simulink model "driveTrain_P_STSMC"  (R2023b)
settings: Solver=VariableStepAuto  StartTime=0.0  StopTime=10.0  RelTol=1e-3
values from neighbouring files (symbols this model uses):
  beta_l = 0.0016    [modelInit_1FT7042.m]
  beta_m = 0.0016    [modelInit_1FT7042.m]
  D_S = 0.0548    [modelInit_1FT7042.m]
  J_l = 1    [modelInit_1FT7042.m]
  J_m = 2.81e-4 + 5.5e-4    (= 0.000831)    [modelInit_1FT7042.m]
  k1 = 4.9905    [modelInit_1FT7042.m]
  k2 = 9.9829    [modelInit_1FT7042.m]
  k_pos = 23.4913    [modelInit_1FT7042.m]
  K_S = 32.94    [modelInit_1FT7042.m]
  N = 1    [modelInit_1FT7042.m]
  T_Cl = 0.0232    [modelInit_1FT7042.m]
  T_Cm = 0.0223    [modelInit_1FT7042.m]
  T_log = 0.001    [modelInit_1FT7042.m]
  T_s = 0.000125    [modelInit_1FT7042.m]
  x_0 = [0,0]    [modelInit_1FT7042.m]
  x_l_0 = [0,0]    [modelInit_1FT7042.m]
  xf = 1    [modelInit_1FT7042.m]
settings Model: Creator=dimpa  LastModifiedBy=s214680
settings DebuggingCC: UnconnectedInputMsg=warning  UnconnectedOutputMsg=warning  UnconnectedLineMsg=warning
settings ModelReferenceCC: EnableRefExpFcnMdlSchedulingChecks=on
settings RTWCC: DLArmComputeVersion=19.05

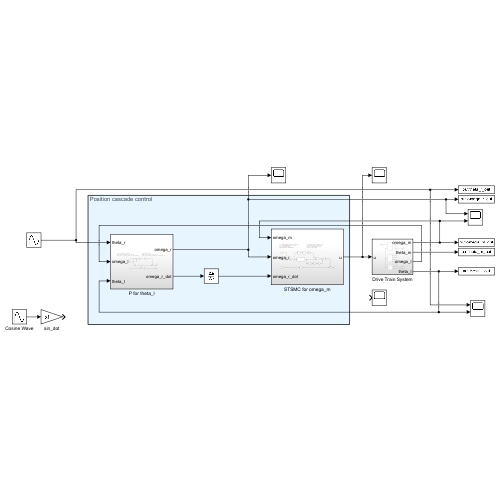
[thumbnail: Simulink's stored preview of the top-level diagram]
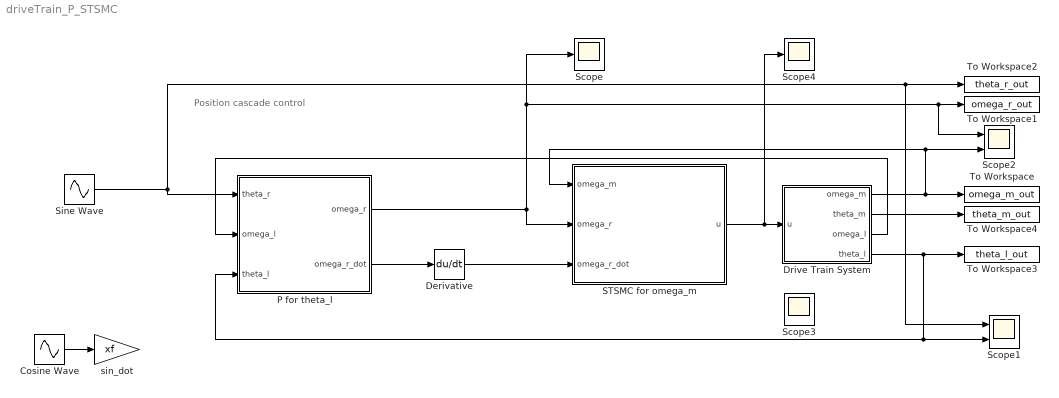
== system driveTrain_P_STSMC ==
  note: Position cascade control
  Cosine Wave : Sin  Frequency=xf  Phase=pi/2  SampleTime=0
  Derivative : Derivative  CoefficientInTFapproximation=1/100
  Drive Train System : Subsystem
  P for theta_l : Subsystem
  STSMC for omega_m : Subsystem
  Scope : Scope
  Scope1 : Scope  NumInputPorts=2
  Scope2 : Scope  NumInputPorts=2
  Scope3 : Scope
  Scope4 : Scope
  Sine Wave : Sin  Frequency=xf  SampleTime=0
  To Workspace : ToWorkspace  VariableName=omega_m_out  SaveFormat=Timeseries  SampleTime=-1
  To Workspace1 : ToWorkspace  VariableName=omega_r_out  SaveFormat=Timeseries  SampleTime=-1
  To Workspace2 : ToWorkspace  VariableName=theta_r_out  SaveFormat=Timeseries  SampleTime=-1
  To Workspace3 : ToWorkspace  VariableName=theta_l_out  SaveFormat=Timeseries  SampleTime=-1
  To Workspace4 : ToWorkspace  VariableName=theta_m_out  SaveFormat=Timeseries  SampleTime=-1
  sin_dot : Gain  Gain=xf
  wires:
  P for theta_l/1(omega_r) -> Scope/1, Scope2/1, To Workspace1/1, STSMC for omega_m/2(omega_r)
  Drive Train System/1(omega_m) -> To Workspace/1, STSMC for omega_m/1(omega_m), Scope2/2
  Drive Train System/4(theta_l) -> To Workspace3/1, P for theta_l/3(theta_l), Scope1/2
  STSMC for omega_m/1(u) -> Drive Train System/1(u), Scope4/1
  Drive Train System/2(theta_m) -> To Workspace4/1
  Drive Train System/3(omega_l) -> P for theta_l/2(omega_l)
  Cosine Wave/1 -> sin_dot/1
  Sine Wave/1 -> Scope1/1, To Workspace2/1, P for theta_l/1(theta_r)
  P for theta_l/2(omega_r_dot) -> Derivative/1
  Derivative/1 -> STSMC for omega_m/3(omega_r_dot)

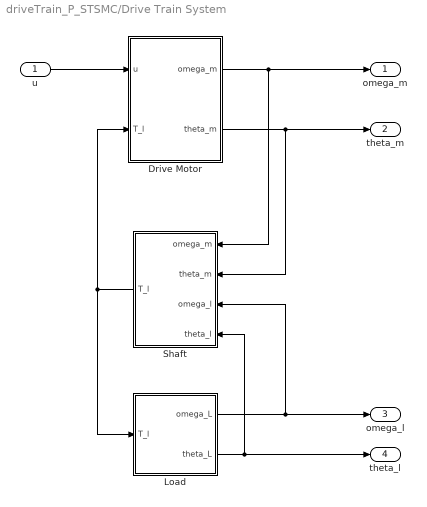
== system driveTrain_P_STSMC/Drive Train System ==
  u : Inport
  Drive Motor : Subsystem
  Load : Subsystem
  Shaft : Subsystem
  omega_m : Outport
  theta_m : Outport  Port=2
  omega_l : Outport  Port=3
  theta_l : Outport  Port=4
  wires:
  Drive Motor/2(theta_m) -> theta_m/1, Shaft/2(theta_m)
  Load/1(omega_L) -> omega_l/1, Shaft/3(omega_l)
  Load/2(theta_L) -> theta_l/1, Shaft/4(theta_l)
  Drive Motor/1(omega_m) -> omega_m/1, Shaft/1(omega_m)
  u/1 -> Drive Motor/1(u)
  Shaft/1(T_l) -> Load/1(T_l), Drive Motor/2(T_l)

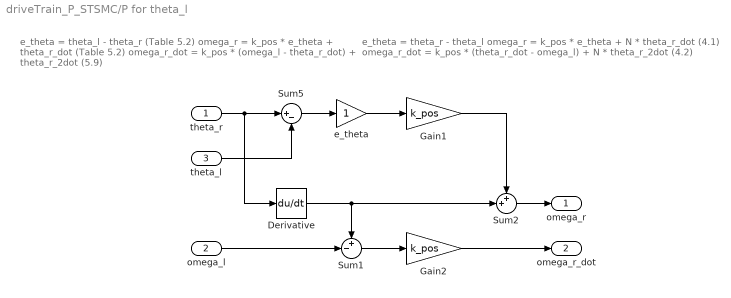
== system driveTrain_P_STSMC/P for theta_l ==
  note: e_theta = theta_l - theta_r (Table 5.2)
      | omega_r = k_pos * e_theta + theta_r_dot (Table 5.2)
      | omega_r_dot = k_pos * (omega_l - theta_r_dot) + theta_r_2dot (5.9)
  note: e_theta = theta_r - theta_l
      | omega_r = k_pos * e_theta + N * theta_r_dot (4.1)
      | omega_r_dot = k_pos * (theta_r_dot - omega_l) + N * theta_r_2dot (4.2)
  theta_r : Inport
  omega_l : Inport  Port=2
  theta_l : Inport  Port=3
  Derivative : Derivative  CoefficientInTFapproximation=1/100
  Gain1 : Gain  Gain=k_pos
  Gain2 : Gain  Gain=k_pos
  Sum1 : Sum  Inputs=+-|
  Sum2 : Sum  Inputs=++|
  Sum5 : Sum  Inputs=|+-
  e_theta : Gain
  omega_r : Outport
  omega_r_dot : Outport  Port=2
  wires:
  Gain2/1 -> omega_r_dot/1
  Sum5/1 -> e_theta/1
  e_theta/1 -> Gain1/1
  theta_r/1 -> Derivative/1, Sum5/1
  theta_l/1 -> Sum5/2
  omega_l/1 -> Sum1/2
  Sum1/1 -> Gain2/1
  Sum2/1 -> omega_r/1
  Gain1/1 -> Sum2/1
  Derivative/1 -> Sum2/2, Sum1/1

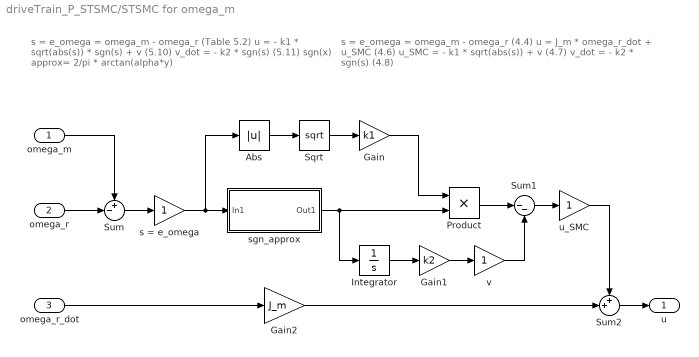
== system driveTrain_P_STSMC/STSMC for omega_m ==
  note: s = e_omega = omega_m - omega_r (Table 5.2)
      | u = - k1 * sqrt(abs(s)) * sgn(s) + v (5.10)
      | v_dot = - k2 * sgn(s) (5.11)
      | sgn(x) approx= 2/pi * arctan(alpha*y)
  note: s = e_omega = omega_m - omega_r (4.4)
      | u = J_m * omega_r_dot + u_SMC (4.6)
      | u_SMC = - k1 * sqrt(abs(s)) + v (4.7)
      | v_dot = - k2 * sgn(s) (4.8)
  omega_m : Inport
  omega_r : Inport  Port=2
  omega_r_dot : Inport  Port=3
  Abs : Abs  SaturateOnIntegerOverflow=off
  Gain : Gain  Gain=k1
  Gain1 : Gain  Gain=k2
  Gain2 : Gain  Gain=J_m
  Integrator : Integrator
  Product : Product
  Sqrt : Sqrt
  Sum : Sum  Inputs=+-|
  Sum1 : Sum  Inputs=|--
  Sum2 : Sum  Inputs=++|
  s = e_omega : Gain
  sgn_approx : Subsystem
  u_SMC : Gain
  v : Gain
  u : Outport
  wires:
  omega_r/1 -> Sum/2
  omega_m/1 -> Sum/1
  Abs/1 -> Sqrt/1
  Sqrt/1 -> Gain/1
  Gain/1 -> Product/1
  sgn_approx/1(Out1) -> Product/2, Integrator/1
  Product/1 -> Sum1/1
  Integrator/1 -> Gain1/1
  Sum2/1 -> u/1
  Gain2/1 -> Sum2/2
  omega_r_dot/1 -> Gain2/1
  Sum/1 -> s = e_omega/1
  s = e_omega/1 -> Abs/1, sgn_approx/1(In1)
  Sum1/1 -> u_SMC/1
  u_SMC/1 -> Sum2/1
  Gain1/1 -> v/1
  v/1 -> Sum1/2

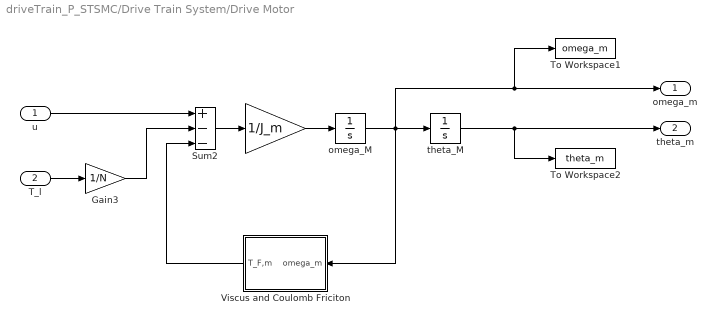
== system driveTrain_P_STSMC/Drive Train System/Drive Motor ==
  u : Inport
  T_l : Inport  Port=2
  "              " : Gain  Gain=1/J_m
  Gain3 : Gain  Gain=1/N
  Sum2 : Sum  Inputs=+--
  To Workspace1 : ToWorkspace  VariableName=omega_m  SaveFormat=Timeseries  SampleTime=T_s
  To Workspace2 : ToWorkspace  VariableName=theta_m  SaveFormat=Timeseries  SampleTime=T_s
  Viscus and Coulomb Friciton : Subsystem
  omega_M : Integrator  InitialCondition=x_0(1)
  theta_M : Integrator  InitialCondition=x_0(2)
  omega_m : Outport
  theta_m : Outport  Port=2
  wires:
  "              "/1 -> omega_M/1
  omega_M/1 -> Viscus and Coulomb Friciton/1(omega_m), theta_M/1, To Workspace1/1, omega_m/1
  u/1 -> Sum2/1
  Sum2/1 -> "              "/1
  theta_M/1 -> To Workspace2/1, theta_m/1
  Viscus and Coulomb Friciton/1(T_F,m) -> Sum2/3
  Gain3/1 -> Sum2/2
  T_l/1 -> Gain3/1

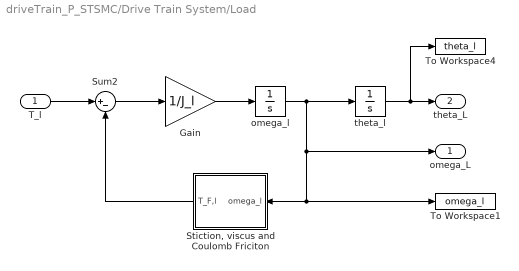
== system driveTrain_P_STSMC/Drive Train System/Load ==
  T_l : Inport
  Gain : Gain  Gain=1/J_l
  "Stiction, viscus and Coulomb Friciton" : Subsystem
  Sum2 : Sum  Inputs=|+-
  To Workspace1 : ToWorkspace  VariableName=omega_l  SaveFormat=Timeseries  SampleTime=T_log
  To Workspace4 : ToWorkspace  VariableName=theta_l  SaveFormat=Timeseries  SampleTime=T_log
  omega_l : Integrator  InitialCondition=x_l_0(1)
  theta_l : Integrator  InitialCondition=x_l_0(2)
  omega_L : Outport
  theta_L : Outport  Port=2
  wires:
  omega_l/1 -> "Stiction, viscus and Coulomb Friciton"/1(omega_l), To Workspace1/1, omega_L/1, theta_l/1
  theta_l/1 -> To Workspace4/1, theta_L/1
  Sum2/1 -> Gain/1
  Gain/1 -> omega_l/1
  T_l/1 -> Sum2/1
  "Stiction, viscus and Coulomb Friciton"/1(T_F,l) -> Sum2/2

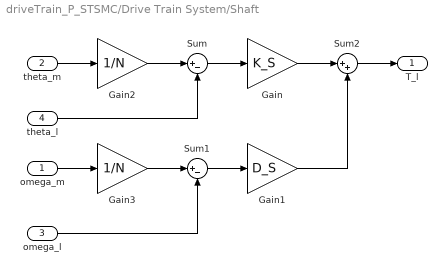
== system driveTrain_P_STSMC/Drive Train System/Shaft ==
  omega_m : Inport
  theta_m : Inport  Port=2
  omega_l : Inport  Port=3
  theta_l : Inport  Port=4
  Gain : Gain  Gain=K_S
  Gain1 : Gain  Gain=D_S
  Gain2 : Gain  Gain=1/N
  Gain3 : Gain  Gain=1/N
  Sum : Sum  Inputs=|+-
  Sum1 : Sum  Inputs=|+-
  Sum2 : Sum  Inputs=|++
  T_l : Outport
  wires:
  theta_m/1 -> Gain2/1
  Gain2/1 -> Sum/1
  theta_l/1 -> Sum/2
  Sum/1 -> Gain/1
  Gain/1 -> Sum2/1
  Gain3/1 -> Sum1/1
  omega_m/1 -> Gain3/1
  omega_l/1 -> Sum1/2
  Sum1/1 -> Gain1/1
  Gain1/1 -> Sum2/2
  Sum2/1 -> T_l/1

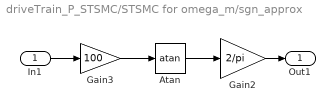
== system driveTrain_P_STSMC/STSMC for omega_m/sgn_approx ==
  In1 : Inport
  Atan : Trigonometry  Operator=atan
  Gain2 : Gain  Gain=2/pi
  Gain3 : Gain  Gain=100
  Out1 : Outport
  wires:
  Gain3/1 -> Atan/1
  Atan/1 -> Gain2/1
  In1/1 -> Gain3/1
  Gain2/1 -> Out1/1

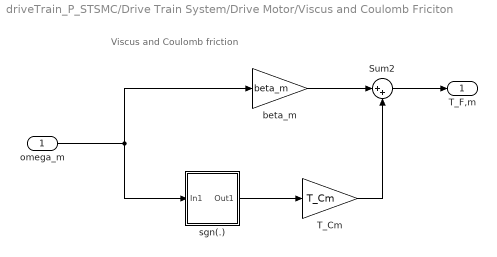
== system driveTrain_P_STSMC/Drive Train System/Drive Motor/Viscus and Coulomb Friciton ==
  note: Viscus and
      | Coulomb friction
  omega_m : Inport
  Sum2 : Sum  Inputs=|++
  T_Cm : Gain  Gain=T_Cm
  beta_m : Gain  Gain=beta_m
  sgn(.) : Subsystem
  T_F,m : Outport
  wires:
  Sum2/1 -> T_F,m/1
  sgn(.)/1(Out1) -> T_Cm/1
  omega_m/1 -> sgn(.)/1(In1), beta_m/1
  T_Cm/1 -> Sum2/2
  beta_m/1 -> Sum2/1

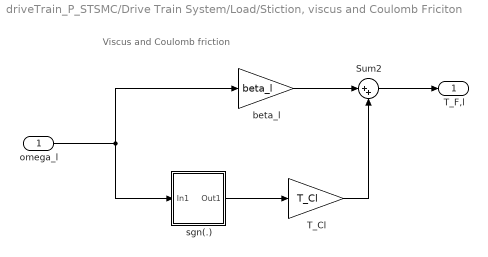
== system driveTrain_P_STSMC/Drive Train System/Load/Stiction, viscus and Coulomb Friciton ==
  note: Viscus and
      | Coulomb friction
  omega_l : Inport
  Sum2 : Sum  Inputs=|++
  T_Cl : Gain  Gain=T_Cl
  beta_l : Gain  Gain=beta_l
  sgn(.) : Subsystem
  T_F,l : Outport
  wires:
  Sum2/1 -> T_F,l/1
  sgn(.)/1(Out1) -> T_Cl/1
  omega_l/1 -> sgn(.)/1(In1), beta_l/1
  T_Cl/1 -> Sum2/2
  beta_l/1 -> Sum2/1

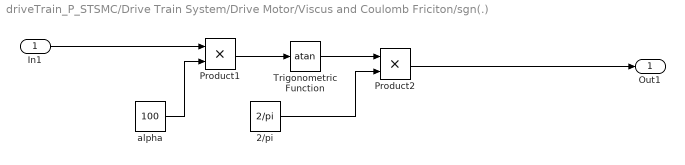
== system driveTrain_P_STSMC/Drive Train System/Drive Motor/Viscus and Coulomb Friciton/sgn(.) ==
  In1 : Inport
  2/pi : Constant  Value=2/pi
  Product1 : Product
  Product2 : Product
  Trigonometric Function : Trigonometry  Operator=atan  SampleTime=T_s
  alpha : Constant  Value=100
  Out1 : Outport
  wires:
  Trigonometric Function/1 -> Product2/1
  Product2/1 -> Out1/1
  In1/1 -> Product1/1
  alpha/1 -> Product1/2
  Product1/1 -> Trigonometric Function/1
  2/pi/1 -> Product2/2

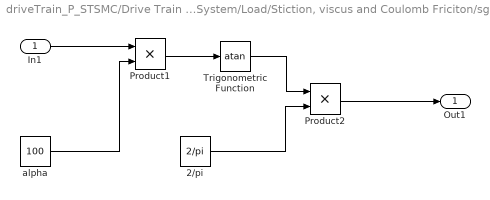
== system driveTrain_P_STSMC/Drive Train System/Load/Stiction, viscus and Coulomb Friciton/sgn(.) ==
  In1 : Inport
  2/pi : Constant  Value=2/pi
  Product1 : Product
  Product2 : Product
  Trigonometric Function : Trigonometry  Operator=atan  SampleTime=T_s
  alpha : Constant  Value=100
  Out1 : Outport
  wires:
  Trigonometric Function/1 -> Product2/1
  Product2/1 -> Out1/1
  In1/1 -> Product1/1
  alpha/1 -> Product1/2
  Product1/1 -> Trigonometric Function/1
  2/pi/1 -> Product2/2
